simulink model "IEEE123_4subsystem"  (R2022b)
settings: Solver=ode4  StartTime=0.0  StopTime=inf  FixedStep=Ts  MaxStep=1e-4  RelTol=1e-3
PreLoadFcn:
  | Ts = 50e-6;
PostLoadFcn:
  | Ts = 50e-6;
InitFcn:
  | %%%%%%%%%%%%%%%%%%%%%%%%
  | % Simulation data for the IEEE 123 Node Test Feeder model
  | %%%%%%%%%%%%%%%%%%%%%%%
  | 
  | % miles/km
  | mi2km = 1.60934;
  | 
  | % feet to km
  | ft2km = 0.0003048;
  | 
  | % microsiemens to Farads
  | ms2F = 1/2/pi/60*1e-6;
  | 
  | %% Configuration 1 - series reactance - ohm/mile
  | 
  | R_1 = [0.4576 0.1560 0.1535;0.1560 0.4666 0.1580;0.1535 0.1580 0.4615];
  | X_1 = [1.0780 0.5017 0.3849;0.5017 1.0482 0.4236;0.3849 0.4236 1.0651];
  | 
  | % charging susceptance - microsiemens/mile
  | 
  | B_1 = [5.6765 -1.8319 -0.6982;-1.8319 5.9809 -1.1645;-0.6982 -1.1645 5.3971];
  | 
  | % convert for SPS
  | 
  | R_1 = R_1/mi2km;
  | 
  | Rs_1=(R_1(1,1)+R_1(2,2)+R_1(3,3))/3;
  | Rm_1=(R_1(1,2)+R_1(1,3)+R_1(2,3))/3;
  | R1_1=Rs_1-Rm_1;
  | R0_1=Rs_1+2*Rm_1;
  | 
  | L_1 = X_1/mi2km/2/pi/60;
  | 
  | Ls_1=(L_1(1,1)+L_1(2,2)+L_1(3,3))/3;
  | Lm_1=(L_1(1,2)+L_1(1,3)+L_1(2,3))/3;
  | L1_1=Ls_1-Lm_1;
  | L0_1=Ls_1+2*Lm_1;
  | 
  | C_1 = B_1/mi2km*ms2F;
  | 
  | Cs_1=(C_1(1,1)+C_1(2,2)+C_1(3,3))/3;
  | Cm_1=(C_1(1,2)+C_1(1,3)+C_1(2,3))/3;
  | C1_1=Cs_1-Cm_1;
  | C0_1=Cs_1+2*Cm_1;
  | 
  | 
  | %% Configuration 2 - series reactance - ohm/mile
  | 
  | R_2 = [0.4666 0.1580 0.1560;0.1580 0.4615 0.1535;0.1560 0.1535 0.4576];
  | X_2 = [1.0482 0.4236 0.5017;0.4236 1.0651 0.3849;0.5017 0.3849 1.0780];
  | 
  | % charging susceptance - microsiemens/mile
  | 
  | B_2 = [5.9809 -1.1645 -1.8319;-1.1645 5.3971 -0.6982;-1.8319 -0.6982 5.6765];
  | 
  | % convert for SPS
  | 
  | R_2 = R_2/mi2km;
  | 
  | Rs_2=(R_2(1,1)+R_2(2,2)+R_2(3,3))/3;
  | ... (+341 lines)
undefined symbols (not defined in the file): D1, Delta, find_system, I, Left, MOV_segment9, powergui, Right, type, V, X
libraries: spsGroundLib x242, spsThreePhaseVIMeasurementLib x134, spsSeriesRLCBranchLib x107, spsSeriesRLCLoadLib x83, spsPiSectionLineLib x61, spsThreePhasePISectionLineLib x60, spsVoltageMeasurementLib x52, spsDCVoltageSourceLib x36, ssn_lib x28, artemis x24, spsACCurrentSourceLib x18, spsOnDelayLib x18
(part 4 of 15)

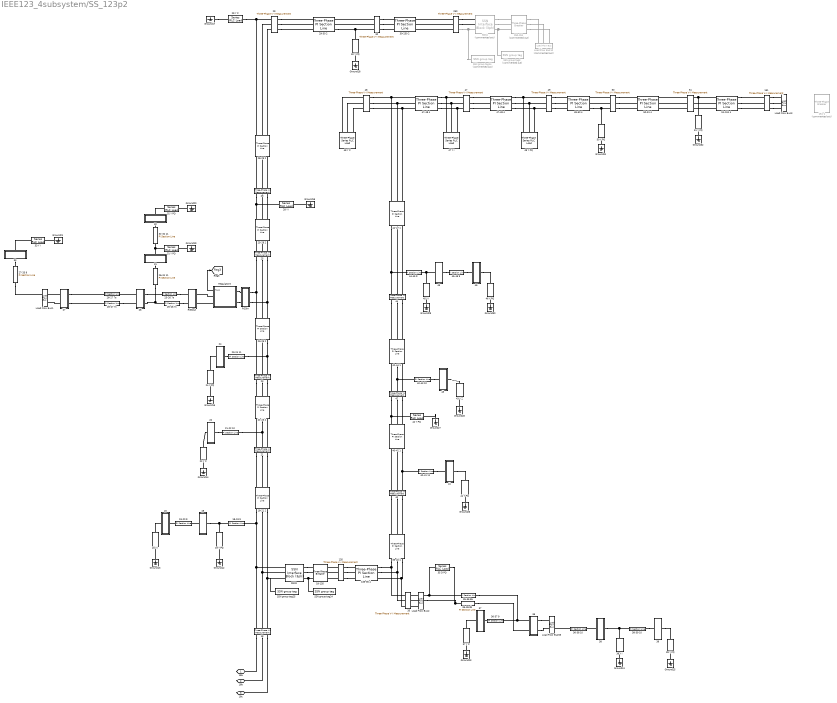
== system IEEE123_4subsystem/SS_123p2 ==
  135 : spsThreePhaseVIMeasurementLib/Three-Phase V-I Measurement  VoltageMeasurement=phase-to-ground  SetLabelV=on  LabelV=V135  Vpu=off  VpuLL=off  CurrentMeasurement=no  SetLabelI=on  LabelI=I800  Ipu=off  Pbase=100e6  Vbase=24900  OutputType=Complex  PhasorSimulation=off  PSBequivalent=0
  135-35 4 : spsThreePhasePISectionLineLib/Three-Phase PI Section Line  LConnTagsString=a|b|c  RConnTagsString=A|B|C  Length=375*ft2km  Frequency=60  Resistances=[R1_4 R0_4]  Inductances=[L1_4 L0_4]  Capacitances=[C1_4 C0_4]
  151 : spsThreePhaseVIMeasurementLib/Three-Phase V-I Measurement  VoltageMeasurement=phase-to-ground  SetLabelV=on  LabelV=V151  Vpu=off  VpuLL=off  CurrentMeasurement=no  SetLabelI=on  LabelI=I65  Ipu=off  Pbase=100e6  Vbase=24900  OutputType=Complex  PhasorSimulation=off  PSBequivalent=0
  151-1 : spsThreePhaseBreakerLib/Three-Phase Breaker  Commented=on  InitialState=open  SwitchA=on  SwitchB=on  SwitchC=on  SwitchTimes="[1/60  5/60]"  External=off  BreakerResistance=0.01  SnubberResistance=1e6  SnubberCapacitance=inf  Measurements=None
  18 : spsThreePhaseVIMeasurementLib/Three-Phase V-I Measurement  VoltageMeasurement=phase-to-ground  SetLabelV=on  LabelV=V18  Vpu=off  VpuLL=off  CurrentMeasurement=yes  SetLabelI=on  LabelI=I18  Ipu=off  Pbase=100e6  Vbase=24900  OutputType=Complex  PhasorSimulation=off  PSBequivalent=0
  18-135 : spsThreePhaseBreakerLib/Three-Phase Breaker  InitialState=closed  SwitchA=on  SwitchB=on  SwitchC=on  SwitchTimes="[1/60  5/60]"  External=off  BreakerResistance=0.01  SnubberResistance=1e6  SnubberCapacitance=inf  Measurements=None
  18-19 9 : spsPiSectionLineLib/Pi Section Line  LConnTagsString=__new0  RConnTagsString=__new0  Phases=1  PiSections=1  Length=250*ft2km  Frequency=60  Resistance=R1_9  Inductance=L1_9  Capacitance=C1_9  SpecifyConductance=off  Conductance=0  Measurements=None  Measurements2=None
      settings: LibrarySourceBlock=sps_lib/Power Grid Elements/Pi Section Line
  18-21 2 : spsThreePhasePISectionLineLib/Three-Phase PI Section Line  LConnTagsString=a|b|c  RConnTagsString=A|B|C  Length=300*ft2km  Frequency=60  Resistances=[R1_2 R0_2]  Inductances=[L1_2 L0_2]  Capacitances=[C1_2 C0_2]
  19 : Subsystem
  19 Y PQ : spsSeriesRLCLoadLib/Series RLC Load  LConnTagsString=a  RConnTagsString=__new0  NominalVoltage=1.0*2401.78  NominalFrequency=60  ActivePower=40e3  InductivePower=20e3  CapacitivePower=0  Setx0=off  InitialVoltage=0  SetiL0=off  InitialCurrent=0  Measurements=None  LoadType=constant PQ
  19-20 9 : spsPiSectionLineLib/Pi Section Line  LConnTagsString=__new0  RConnTagsString=__new0  Phases=1  PiSections=1  Length=325*ft2km  Frequency=60  Resistance=R1_9  Inductance=L1_9  Capacitance=C1_9  SpecifyConductance=off  Conductance=0  Measurements=None  Measurements2=None
      settings: LibrarySourceBlock=sps_lib/Power Grid Elements/Pi Section Line
  20 : Subsystem
  20 Y I : spsSeriesRLCLoadLib/Series RLC Load  LConnTagsString=a  RConnTagsString=__new0  NominalVoltage=1.0*2401.78  NominalFrequency=60  ActivePower=40e3  InductivePower=20e3  CapacitivePower=0  Setx0=off  InitialVoltage=0  SetiL0=off  InitialCurrent=0  Measurements=None  LoadType=constant I
  21 : spsThreePhaseVIMeasurementLib/Three-Phase V-I Measurement  VoltageMeasurement=phase-to-ground  SetLabelV=on  LabelV=V21  Vpu=off  VpuLL=off  CurrentMeasurement=yes  SetLabelI=on  LabelI=I21  Ipu=off  Pbase=100e6  Vbase=24900  OutputType=Complex  PhasorSimulation=off  PSBequivalent=0
  21-22 10 : spsPiSectionLineLib/Pi Section Line  LConnTagsString=__new0  RConnTagsString=__new0  Phases=1  PiSections=1  Length=525*ft2km  Frequency=60  Resistance=R1_10  Inductance=L1_10  Capacitance=C1_10  SpecifyConductance=off  Conductance=0  Measurements=None  Measurements2=None
      settings: LibrarySourceBlock=sps_lib/Power Grid Elements/Pi Section Line
  21-23 2 : spsThreePhasePISectionLineLib/Three-Phase PI Section Line  LConnTagsString=a|b|c  RConnTagsString=A|B|C  Length=250*ft2km  Frequency=60  Resistances=[R1_2 R0_2]  Inductances=[L1_2 L0_2]  Capacitances=[C1_2 C0_2]
  22 : Subsystem
  22 Y Z : spsSeriesRLCLoadLib/Series RLC Load  LConnTagsString=a  RConnTagsString=__new0  NominalVoltage=1.0*2401.78  NominalFrequency=60  ActivePower=40e3  InductivePower=20e3  CapacitivePower=0  Setx0=off  InitialVoltage=0  SetiL0=off  InitialCurrent=0  Measurements=None  LoadType=constant Z
  23 : spsThreePhaseVIMeasurementLib/Three-Phase V-I Measurement  VoltageMeasurement=phase-to-ground  SetLabelV=on  LabelV=V23  Vpu=off  VpuLL=off  CurrentMeasurement=no  SetLabelI=on  LabelI=I800  Ipu=off  Pbase=100e6  Vbase=24900  OutputType=Complex  PhasorSimulation=off  PSBequivalent=0
  23-24 11 : spsPiSectionLineLib/Pi Section Line  LConnTagsString=__new0  RConnTagsString=__new0  Phases=1  PiSections=1  Length=550*ft2km  Frequency=60  Resistance=R1_11  Inductance=L1_11  Capacitance=C1_11  SpecifyConductance=off  Conductance=0  Measurements=None  Measurements2=None
      settings: LibrarySourceBlock=sps_lib/Power Grid Elements/Pi Section Line
  23-25 2 : spsThreePhasePISectionLineLib/Three-Phase PI Section Line  LConnTagsString=a|b|c  RConnTagsString=A|B|C  Length=275*ft2km  Frequency=60  Resistances=[R1_2 R0_2]  Inductances=[L1_2 L0_2]  Capacitances=[C1_2 C0_2]
  24 : Subsystem
  24 Y PQ : spsSeriesRLCLoadLib/Series RLC Load  LConnTagsString=a  RConnTagsString=__new0  NominalVoltage=1.0*2401.78  NominalFrequency=60  ActivePower=40e3  InductivePower=20e3  CapacitivePower=0  Setx0=off  InitialVoltage=0  SetiL0=off  InitialCurrent=0  Measurements=None  LoadType=constant PQ
  25 : spsThreePhaseVIMeasurementLib/Three-Phase V-I Measurement  VoltageMeasurement=phase-to-ground  SetLabelV=on  LabelV=V25  Vpu=off  VpuLL=off  CurrentMeasurement=no  SetLabelI=on  LabelI=I800  Ipu=off  Pbase=100e6  Vbase=24900  OutputType=Complex  PhasorSimulation=off  PSBequivalent=0
  25-26 7a : spsPiSectionLineLib/Pi Section Line  LConnTagsString=__new0  RConnTagsString=__new0  Phases=1  PiSections=1  Length=350*ft2km  Frequency=60  Resistance=R1_7  Inductance=L1_7  Capacitance=C1_7  SpecifyConductance=off  Conductance=0  Measurements=None  Measurements2=None
      settings: LibrarySourceBlock=sps_lib/Power Grid Elements/Pi Section Line
  25-26 7c : spsPiSectionLineLib/Pi Section Line  LConnTagsString=__new0  RConnTagsString=__new0  Phases=1  PiSections=1  Length=350*ft2km  Frequency=60  Resistance=R1_7  Inductance=L1_7  Capacitance=C1_7  SpecifyConductance=off  Conductance=0  Measurements=None  Measurements2=None
      settings: LibrarySourceBlock=sps_lib/Power Grid Elements/Pi Section Line
  25-28 2 : spsThreePhasePISectionLineLib/Three-Phase PI Section Line  LConnTagsString=a|b|c  RConnTagsString=A|B|C  Length=200*ft2km  Frequency=60  Resistances=[R1_2 R0_2]  Inductances=[L1_2 L0_2]  Capacitances=[C1_2 C0_2]
  250 : spsThreePhaseVIMeasurementLib/Three-Phase V-I Measurement  VoltageMeasurement=phase-to-ground  SetLabelV=on  LabelV=V250  Vpu=off  VpuLL=off  CurrentMeasurement=no  SetLabelI=on  LabelI=I800  Ipu=off  Pbase=100e6  Vbase=24900  OutputType=Complex  PhasorSimulation=off  PSBequivalent=0
  250-251 : spsThreePhaseBreakerLib/Three-Phase Breaker  Commented=on  InitialState=open  SwitchA=on  SwitchB=on  SwitchC=on  SwitchTimes="[1/60  5/60]"  External=off  BreakerResistance=0.01  SnubberResistance=1e6  SnubberCapacitance=inf  Measurements=None
  26 : Subsystem
  26-27 7a : spsPiSectionLineLib/Pi Section Line  LConnTagsString=__new0  RConnTagsString=__new0  Phases=1  PiSections=1  Length=275*ft2km  Frequency=60  Resistance=R1_7  Inductance=L1_7  Capacitance=C1_7  SpecifyConductance=off  Conductance=0  Measurements=None  Measurements2=None
      settings: LibrarySourceBlock=sps_lib/Power Grid Elements/Pi Section Line
  26-27 7c : spsPiSectionLineLib/Pi Section Line  LConnTagsString=__new0  RConnTagsString=__new0  Phases=1  PiSections=1  Length=275*ft2km  Frequency=60  Resistance=R1_7  Inductance=L1_7  Capacitance=C1_7  SpecifyConductance=off  Conductance=0  Measurements=None  Measurements2=None
      settings: LibrarySourceBlock=sps_lib/Power Grid Elements/Pi Section Line
  26-31 11 : spsPiSectionLineLib/Pi Section Line  LConnTagsString=__new0  RConnTagsString=__new0  Phases=1  PiSections=1  Length=225*ft2km  Frequency=60  Resistance=R1_11  Inductance=L1_11  Capacitance=C1_11  SpecifyConductance=off  Conductance=0  Measurements=None  Measurements2=None
      settings: LibrarySourceBlock=sps_lib/Power Grid Elements/Pi Section Line
  27 : Subsystem
  27-33 9 : spsPiSectionLineLib/Pi Section Line  LConnTagsString=__new0  RConnTagsString=__new0  Phases=1  PiSections=1  Length=500*ft2km  Frequency=60  Resistance=R1_9  Inductance=L1_9  Capacitance=C1_9  SpecifyConductance=off  Conductance=0  Measurements=None  Measurements2=None
      settings: LibrarySourceBlock=sps_lib/Power Grid Elements/Pi Section Line
  28 : spsThreePhaseVIMeasurementLib/Three-Phase V-I Measurement  VoltageMeasurement=phase-to-ground  SetLabelV=on  LabelV=V28  Vpu=off  VpuLL=off  CurrentMeasurement=no  SetLabelI=on  LabelI=I800  Ipu=off  Pbase=100e6  Vbase=24900  OutputType=Complex  PhasorSimulation=off  PSBequivalent=0
  28 Y I : spsSeriesRLCLoadLib/Series RLC Load  LConnTagsString=a  RConnTagsString=__new0  NominalVoltage=1.0*2401.78  NominalFrequency=60  ActivePower=40e3  InductivePower=20e3  CapacitivePower=0  Setx0=off  InitialVoltage=0  SetiL0=off  InitialCurrent=0  Measurements=None  LoadType=constant I
  28-29 2 : spsThreePhasePISectionLineLib/Three-Phase PI Section Line  LConnTagsString=a|b|c  RConnTagsString=A|B|C  Length=300*ft2km  Frequency=60  Resistances=[R1_2 R0_2]  Inductances=[L1_2 L0_2]  Capacitances=[C1_2 C0_2]
  29 : spsThreePhaseVIMeasurementLib/Three-Phase V-I Measurement  VoltageMeasurement=phase-to-ground  SetLabelV=on  LabelV=V29  Vpu=off  VpuLL=off  CurrentMeasurement=no  SetLabelI=on  LabelI=I800  Ipu=off  Pbase=100e6  Vbase=24900  OutputType=Complex  PhasorSimulation=off  PSBequivalent=0
  29 Y Z : spsSeriesRLCLoadLib/Series RLC Load  LConnTagsString=a  RConnTagsString=__new0  NominalVoltage=1.0*2401.78  NominalFrequency=60  ActivePower=40e3  InductivePower=20e3  CapacitivePower=0  Setx0=off  InitialVoltage=0  SetiL0=off  InitialCurrent=0  Measurements=None  LoadType=constant Z
  29-30 2 : spsThreePhasePISectionLineLib/Three-Phase PI Section Line  LConnTagsString=a|b|c  RConnTagsString=A|B|C  Length=350*ft2km  Frequency=60  Resistances=[R1_2 R0_2]  Inductances=[L1_2 L0_2]  Capacitances=[C1_2 C0_2]
  "30 " : spsThreePhaseVIMeasurementLib/Three-Phase V-I Measurement  VoltageMeasurement=phase-to-ground  SetLabelV=on  LabelV=V30  Vpu=off  VpuLL=off  CurrentMeasurement=no  SetLabelI=on  LabelI=I800  Ipu=off  Pbase=100e6  Vbase=24900  OutputType=Complex  PhasorSimulation=off  PSBequivalent=0
  30 Y PQ : spsSeriesRLCLoadLib/Series RLC Load  LConnTagsString=a  RConnTagsString=__new0  NominalVoltage=1.0*2401.78  NominalFrequency=60  ActivePower=40e3  InductivePower=20e3  CapacitivePower=0  Setx0=off  InitialVoltage=0  SetiL0=off  InitialCurrent=0  Measurements=None  LoadType=constant PQ
  30-250 2 : spsThreePhasePISectionLineLib/Three-Phase PI Section Line  LConnTagsString=a|b|c  RConnTagsString=A|B|C  Length=200*ft2km  Frequency=60  Resistances=[R1_2 R0_2]  Inductances=[L1_2 L0_2]  Capacitances=[C1_2 C0_2]
  31 : Subsystem
  31 Y PQ : spsSeriesRLCLoadLib/Series RLC Load  LConnTagsString=a  RConnTagsString=__new0  NominalVoltage=1.0*2401.78  NominalFrequency=60  ActivePower=20e3  InductivePower=10e3  CapacitivePower=0  Setx0=off  InitialVoltage=0  SetiL0=off  InitialCurrent=0  Measurements=None  LoadType=constant PQ
  31-32 11 : spsPiSectionLineLib/Pi Section Line  LConnTagsString=__new0  RConnTagsString=__new0  Phases=1  PiSections=1  Length=300*ft2km  Frequency=60  Resistance=R1_11  Inductance=L1_11  Capacitance=C1_11  SpecifyConductance=off  Conductance=0  Measurements=None  Measurements2=None
      settings: LibrarySourceBlock=sps_lib/Power Grid Elements/Pi Section Line
  32 : Subsystem
  32 Y PQ : spsSeriesRLCLoadLib/Series RLC Load  LConnTagsString=a  RConnTagsString=__new0  NominalVoltage=1.0*2401.78  NominalFrequency=60  ActivePower=20e3  InductivePower=10e3  CapacitivePower=0  Setx0=off  InitialVoltage=0  SetiL0=off  InitialCurrent=0  Measurements=None  LoadType=constant PQ
  33 : Subsystem
  33 Y I : spsSeriesRLCLoadLib/Series RLC Load  LConnTagsString=a  RConnTagsString=__new0  NominalVoltage=1.0*2401.78  NominalFrequency=60  ActivePower=40e3  InductivePower=20e3  CapacitivePower=0  Setx0=off  InitialVoltage=0  SetiL0=off  InitialCurrent=0  Measurements=None  LoadType=constant I
  35 : spsThreePhaseVIMeasurementLib/Three-Phase V-I Measurement  VoltageMeasurement=phase-to-ground  SetLabelV=on  LabelV=V35  Vpu=off  VpuLL=off  CurrentMeasurement=no  SetLabelI=on  LabelI=I800  Ipu=off  Pbase=100e6  Vbase=24900  OutputType=Complex  PhasorSimulation=off  PSBequivalent=0
  35 D PQ : spsSeriesRLCLoadLib/Series RLC Load  LConnTagsString=a  RConnTagsString=__new0  NominalVoltage=1.0*4160  NominalFrequency=60  ActivePower=40e3  InductivePower=20e3  CapacitivePower=0  Setx0=off  InitialVoltage=0  SetiL0=off  InitialCurrent=0  Measurements=None  LoadType=constant I
  35-36 8a : spsPiSectionLineLib/Pi Section Line  LConnTagsString=__new0  RConnTagsString=__new0  Phases=1  PiSections=1  Length=650*ft2km  Frequency=60  Resistance=R1_8  Inductance=L1_8  Capacitance=C1_8  SpecifyConductance=off  Conductance=0  Measurements=None  Measurements2=None
      settings: LibrarySourceBlock=sps_lib/Power Grid Elements/Pi Section Line
  35-36 8b : spsPiSectionLineLib/Pi Section Line  LConnTagsString=__new0  RConnTagsString=__new0  Phases=1  PiSections=1  Length=650*ft2km  Frequency=60  Resistance=R1_8  Inductance=L1_8  Capacitance=C1_8  SpecifyConductance=off  Conductance=0  Measurements=None  Measurements2=None
      settings: LibrarySourceBlock=sps_lib/Power Grid Elements/Pi Section Line
  35-40 1 : spsThreePhasePISectionLineLib/Three-Phase PI Section Line  LConnTagsString=a|b|c  RConnTagsString=A|B|C  Length=250*ft2km  Frequency=60  Resistances=[R1_1 R0_1]  Inductances=[L1_1 L0_1]  Capacitances=[C1_1 C0_1]
  36 : Subsystem
  36-37 9 : spsPiSectionLineLib/Pi Section Line  LConnTagsString=__new0  RConnTagsString=__new0  Phases=1  PiSections=1  Length=300*ft2km  Frequency=60  Resistance=R1_9  Inductance=L1_9  Capacitance=C1_9  SpecifyConductance=off  Conductance=0  Measurements=None  Measurements2=None
      settings: LibrarySourceBlock=sps_lib/Power Grid Elements/Pi Section Line
  36-38 10 : spsPiSectionLineLib/Pi Section Line  LConnTagsString=__new0  RConnTagsString=__new0  Phases=1  PiSections=1  Length=250*ft2km  Frequency=60  Resistance=R1_10  Inductance=L1_10  Capacitance=C1_10  SpecifyConductance=off  Conductance=0  Measurements=None  Measurements2=None
      settings: LibrarySourceBlock=sps_lib/Power Grid Elements/Pi Section Line
  37 : Subsystem
  37 Y Z : spsSeriesRLCLoadLib/Series RLC Load  LConnTagsString=a  RConnTagsString=__new0  NominalVoltage=1.0*2401.78  NominalFrequency=60  ActivePower=40e3  InductivePower=20e3  CapacitivePower=0  Setx0=off  InitialVoltage=0  SetiL0=off  InitialCurrent=0  Measurements=None  LoadType=constant Z
  38 : Subsystem
  38 Y I : spsSeriesRLCLoadLib/Series RLC Load  LConnTagsString=a  RConnTagsString=__new0  NominalVoltage=1.0*2401.78  NominalFrequency=60  ActivePower=20e3  InductivePower=10e3  CapacitivePower=0  Setx0=off  InitialVoltage=0  SetiL0=off  InitialCurrent=0  Measurements=None  LoadType=constant I
  38-39 10 : spsPiSectionLineLib/Pi Section Line  LConnTagsString=__new0  RConnTagsString=__new0  Phases=1  PiSections=1  Length=325*ft2km  Frequency=60  Resistance=R1_10  Inductance=L1_10  Capacitance=C1_10  SpecifyConductance=off  Conductance=0  Measurements=None  Measurements2=None
      settings: LibrarySourceBlock=sps_lib/Power Grid Elements/Pi Section Line
  39 : Subsystem
  39 Y PQ : spsSeriesRLCLoadLib/Series RLC Load  LConnTagsString=a  RConnTagsString=__new0  NominalVoltage=1.0*2401.78  NominalFrequency=60  ActivePower=20e3  InductivePower=10e3  CapacitivePower=0  Setx0=off  InitialVoltage=0  SetiL0=off  InitialCurrent=0  Measurements=None  LoadType=constant PQ
  40 : spsThreePhaseVIMeasurementLib/Three-Phase V-I Measurement  VoltageMeasurement=phase-to-ground  SetLabelV=on  LabelV=V40  Vpu=off  VpuLL=off  CurrentMeasurement=no  SetLabelI=on  LabelI=I800  Ipu=off  Pbase=100e6  Vbase=24900  OutputType=Complex  PhasorSimulation=off  PSBequivalent=0
  40-41 11 : spsPiSectionLineLib/Pi Section Line  LConnTagsString=__new0  RConnTagsString=__new0  Phases=1  PiSections=1  Length=325*ft2km  Frequency=60  Resistance=R1_11  Inductance=L1_11  Capacitance=C1_11  SpecifyConductance=off  Conductance=0  Measurements=None  Measurements2=None
      settings: LibrarySourceBlock=sps_lib/Power Grid Elements/Pi Section Line
  40-42 1 : spsThreePhasePISectionLineLib/Three-Phase PI Section Line  LConnTagsString=a|b|c  RConnTagsString=A|B|C  Length=250*ft2km  Frequency=60  Resistances=[R1_1 R0_1]  Inductances=[L1_1 L0_1]  Capacitances=[C1_1 C0_1]
  41 : Subsystem
  41 Y PQ : spsSeriesRLCLoadLib/Series RLC Load  LConnTagsString=a  RConnTagsString=__new0  NominalVoltage=1.0*2401.78  NominalFrequency=60  ActivePower=20e3  InductivePower=10e3  CapacitivePower=0  Setx0=off  InitialVoltage=0  SetiL0=off  InitialCurrent=0  Measurements=None  LoadType=constant PQ
  42 : spsThreePhaseVIMeasurementLib/Three-Phase V-I Measurement  VoltageMeasurement=phase-to-ground  SetLabelV=on  LabelV=V42  Vpu=off  VpuLL=off  CurrentMeasurement=no  SetLabelI=on  LabelI=I800  Ipu=off  Pbase=100e6  Vbase=24900  OutputType=Complex  PhasorSimulation=off  PSBequivalent=0
  42 Y PQ : spsSeriesRLCLoadLib/Series RLC Load  LConnTagsString=a  RConnTagsString=__new0  NominalVoltage=1.0*2401.78  NominalFrequency=60  ActivePower=20e3  InductivePower=10e3  CapacitivePower=0  Setx0=off  InitialVoltage=0  SetiL0=off  InitialCurrent=0  Measurements=None  LoadType=constant PQ
  42-43 10 : spsPiSectionLineLib/Pi Section Line  LConnTagsString=__new0  RConnTagsString=__new0  Phases=1  PiSections=1  Length=500*ft2km  Frequency=60  Resistance=R1_10  Inductance=L1_10  Capacitance=C1_10  SpecifyConductance=off  Conductance=0  Measurements=None  Measurements2=None
      settings: LibrarySourceBlock=sps_lib/Power Grid Elements/Pi Section Line
  42-44 1 : spsThreePhasePISectionLineLib/Three-Phase PI Section Line  LConnTagsString=a|b|c  RConnTagsString=A|B|C  Length=200*ft2km  Frequency=60  Resistances=[R1_1 R0_1]  Inductances=[L1_1 L0_1]  Capacitances=[C1_1 C0_1]
  43 : Subsystem
  43 Y Z : spsSeriesRLCLoadLib/Series RLC Load  LConnTagsString=a  RConnTagsString=__new0  NominalVoltage=1.0*2401.78  NominalFrequency=60  ActivePower=40e3  InductivePower=20e3  CapacitivePower=0  Setx0=off  InitialVoltage=0  SetiL0=off  InitialCurrent=0  Measurements=None  LoadType=constant Z
  44 : spsThreePhaseVIMeasurementLib/Three-Phase V-I Measurement  VoltageMeasurement=phase-to-ground  SetLabelV=on  LabelV=V44  Vpu=off  VpuLL=off  CurrentMeasurement=no  SetLabelI=on  LabelI=I800  Ipu=off  Pbase=100e6  Vbase=24900  OutputType=Complex  PhasorSimulation=off  PSBequivalent=0
  44-45 9 : spsPiSectionLineLib/Pi Section Line  LConnTagsString=__new0  RConnTagsString=__new0  Phases=1  PiSections=1  Length=200*ft2km  Frequency=60  Resistance=R1_9  Inductance=L1_9  Capacitance=C1_9  SpecifyConductance=off  Conductance=0  Measurements=None  Measurements2=None
      settings: LibrarySourceBlock=sps_lib/Power Grid Elements/Pi Section Line
  44-47 1 : spsThreePhasePISectionLineLib/Three-Phase PI Section Line  LConnTagsString=a|b|c  RConnTagsString=A|B|C  Length=250*ft2km  Frequency=60  Resistances=[R1_1 R0_1]  Inductances=[L1_1 L0_1]  Capacitances=[C1_1 C0_1]
  45 : Subsystem
  45 Y I : spsSeriesRLCLoadLib/Series RLC Load  LConnTagsString=a  RConnTagsString=__new0  NominalVoltage=1.0*2401.78  NominalFrequency=60  ActivePower=20e3  InductivePower=10e3  CapacitivePower=0  Setx0=off  InitialVoltage=0  SetiL0=off  InitialCurrent=0  Measurements=None  LoadType=constant I
  45-46 9 : spsPiSectionLineLib/Pi Section Line  LConnTagsString=__new0  RConnTagsString=__new0  Phases=1  PiSections=1  Length=300*ft2km  Frequency=60  Resistance=R1_9  Inductance=L1_9  Capacitance=C1_9  SpecifyConductance=off  Conductance=0  Measurements=None  Measurements2=None
      settings: LibrarySourceBlock=sps_lib/Power Grid Elements/Pi Section Line
  46 : Subsystem
  46 Y PQ : spsSeriesRLCLoadLib/Series RLC Load  LConnTagsString=a  RConnTagsString=__new0  NominalVoltage=1.0*2401.78  NominalFrequency=60  ActivePower=20e3  InductivePower=10e3  CapacitivePower=0  Setx0=off  InitialVoltage=0  SetiL0=off  InitialCurrent=0  Measurements=None  LoadType=constant PQ
  47 : spsThreePhaseVIMeasurementLib/Three-Phase V-I Measurement  VoltageMeasurement=phase-to-ground  SetLabelV=on  LabelV=V47  Vpu=off  VpuLL=off  CurrentMeasurement=no  SetLabelI=on  LabelI=I800  Ipu=off  Pbase=100e6  Vbase=24900  OutputType=Complex  PhasorSimulation=off  PSBequivalent=0
  47 Y I : spsThreePhaseSeriesRLCLoadLib/Three-Phase Series RLC Load  LConnTagsString=A|B|C  Configuration=Y (grounded)  NominalVoltage=120e3  Vabc=[ 1.0 1.0 1.0]*2401.78  Vabcp=[1e3 1e3 1e3]  NominalFrequency=60  UnbalancedPower=on  ActivePower=1e+006  InductivePower=0  CapacitivePower=0  Pabc=[35 35 35 ]*1e3  QLabc=[25 25 25 ]*1e3  QCabc=[0 0 0]  Pabcp=[10e3 9e3 11e3]  QLabcp=[100 90 110]  QCabcp=[100 90 110]  Measurements=None  LoadType=constant I
  47-48 4 : spsThreePhasePISectionLineLib/Three-Phase PI Section Line  LConnTagsString=a|b|c  RConnTagsString=A|B|C  Length=150*ft2km  Frequency=60  Resistances=[R1_4 R0_4]  Inductances=[L1_4 L0_4]  Capacitances=[C1_4 C0_4]
  47-49 4 : spsThreePhasePISectionLineLib/Three-Phase PI Section Line  LConnTagsString=a|b|c  RConnTagsString=A|B|C  Length=250*ft2km  Frequency=60  Resistances=[R1_4 R0_4]  Inductances=[L1_4 L0_4]  Capacitances=[C1_4 C0_4]
  48 : spsThreePhaseVIMeasurementLib/Three-Phase V-I Measurement  VoltageMeasurement=phase-to-ground  SetLabelV=on  LabelV=V48  Vpu=off  VpuLL=off  CurrentMeasurement=no  SetLabelI=on  LabelI=I800  Ipu=off  Pbase=100e6  Vbase=24900  OutputType=Complex  PhasorSimulation=off  PSBequivalent=0
  48 Y Z : spsThreePhaseSeriesRLCLoadLib/Three-Phase Series RLC Load  LConnTagsString=A|B|C  Configuration=Y (grounded)  NominalVoltage=120e3  Vabc=[ 1.0 1.0 1.0]*2401.78  Vabcp=[1e3 1e3 1e3]  NominalFrequency=60  UnbalancedPower=on  ActivePower=1e+006  InductivePower=0  CapacitivePower=0  Pabc=[70 70 70]*1e3  QLabc=[50 50 50]*1e3  QCabc=[0 0 0]  Pabcp=[10e3 9e3 11e3]  QLabcp=[100 90 110]  QCabcp=[100 90 110]  Measurements=None  LoadType=constant Z
  49 : spsThreePhaseVIMeasurementLib/Three-Phase V-I Measurement  VoltageMeasurement=phase-to-ground  SetLabelV=on  LabelV=V49  Vpu=off  VpuLL=off  CurrentMeasurement=no  SetLabelI=on  LabelI=I800  Ipu=off  Pbase=100e6  Vbase=24900  OutputType=Complex  PhasorSimulation=off  PSBequivalent=0
  49 Y PQ : spsThreePhaseSeriesRLCLoadLib/Three-Phase Series RLC Load  LConnTagsString=A|B|C  Configuration=Y (grounded)  NominalVoltage=120e3  Vabc=[ 1.0 1.0 1.0]*2401.78  Vabcp=[1e3 1e3 1e3]  NominalFrequency=60  UnbalancedPower=on  ActivePower=1e+006  InductivePower=0  CapacitivePower=0  Pabc=[35 70 35]*1e3  QLabc=[25 50 20]*1e3  QCabc=[0 0 0]  Pabcp=[10e3 9e3 11e3]  QLabcp=[100 90 110]  QCabcp=[100 90 110]  Measurements=None  LoadType=constant PQ
  49-50 4 : spsThreePhasePISectionLineLib/Three-Phase PI Section Line  LConnTagsString=a|b|c  RConnTagsString=A|B|C  Length=250*ft2km  Frequency=60  Resistances=[R1_4 R0_4]  Inductances=[L1_4 L0_4]  Capacitances=[C1_4 C0_4]
  50 : spsThreePhaseVIMeasurementLib/Three-Phase V-I Measurement  VoltageMeasurement=phase-to-ground  SetLabelV=on  LabelV=V50  Vpu=off  VpuLL=off  CurrentMeasurement=no  SetLabelI=on  LabelI=I800  Ipu=off  Pbase=100e6  Vbase=24900  OutputType=Complex  PhasorSimulation=off  PSBequivalent=0
  50 Y PQ : spsSeriesRLCLoadLib/Series RLC Load  LConnTagsString=a  RConnTagsString=__new0  NominalVoltage=1.0*2401.78  NominalFrequency=60  ActivePower=40e3  InductivePower=20e3  CapacitivePower=0  Setx0=off  InitialVoltage=0  SetiL0=off  InitialCurrent=0  Measurements=None  LoadType=constant PQ
  50-51 4 : spsThreePhasePISectionLineLib/Three-Phase PI Section Line  LConnTagsString=a|b|c  RConnTagsString=A|B|C  Length=250*ft2km  Frequency=60  Resistances=[R1_4 R0_4]  Inductances=[L1_4 L0_4]  Capacitances=[C1_4 C0_4]
  51 : spsThreePhaseVIMeasurementLib/Three-Phase V-I Measurement  VoltageMeasurement=phase-to-ground  SetLabelV=on  LabelV=V51  Vpu=off  VpuLL=off  CurrentMeasurement=no  SetLabelI=on  LabelI=I800  Ipu=off  Pbase=100e6  Vbase=24900  OutputType=Complex  PhasorSimulation=off  PSBequivalent=0
  51 Y PQ : spsSeriesRLCLoadLib/Series RLC Load  LConnTagsString=a  RConnTagsString=__new0  NominalVoltage=1.0*2401.78  NominalFrequency=60  ActivePower=20e3  InductivePower=10e3  CapacitivePower=0  Setx0=off  InitialVoltage=0  SetiL0=off  InitialCurrent=0  Measurements=None  LoadType=constant PQ
  51-151 4 : spsThreePhasePISectionLineLib/Three-Phase PI Section Line  LConnTagsString=a|b|c  RConnTagsString=A|B|C  Length=500*ft2km  Frequency=60  Resistances=[R1_4 R0_4]  Inductances=[L1_4 L0_4]  Capacitances=[C1_4 C0_4]
  Ground{12..21,23..32} (20 alike) : spsGroundLib/Ground  LConnTagsString=a
  Load Flow Bus1 : spsLoadFlowBusLib/Load Flow Bus  LConnTagsString=a|b  RConnTagsString=a|b  Phases=AC  Connectors=on both sides  ID=27  Vbase=4160/sqrt(3)  Vref=[1.0 1.0]  Vangle=[0 120]  VLF=1  VLFb=1  VLFc=1  angleLF=0  angleLFb=0  angleLFc=0
  Load Flow Bus10 : spsLoadFlowBusLib/Load Flow Bus  Commented=on  LConnTagsString=a|b|c  Phases=ABC  Connectors=on one side  ID=251  Vbase=4160/sqrt(3)  Vref=[1.0 1.0 1.0]  Vangle=[0 -120 120]  VLF=1  VLFb=1  VLFc=1  angleLF=0  angleLFb=0  angleLFc=0
  Load Flow Bus2 : spsLoadFlowBusLib/Load Flow Bus  LConnTagsString=a|b|c  RConnTagsString=a|b|c  Phases=ABC  Connectors=on both sides  ID=36  Vbase=4160/sqrt(3)  Vref=[1.0 1.0]  Vangle=[0 -120]  VLF=1  VLFb=1  VLFc=1  angleLF=0  angleLFb=0  angleLFc=0
  Load Flow Bus3 : spsLoadFlowBusLib/Load Flow Bus  LConnTagsString=a|b|c  Phases=ABC  Connectors=on one side  ID=150  Vbase=4160/sqrt(3)  Vref=[1.0 1.0 1.0]  Vangle=[0 -120 120]  VLF=1  VLFb=1  VLFc=1  angleLF=0  angleLFb=0  angleLFc=0
  Load Flow Bus55 : spsLoadFlowBusLib/Load Flow Bus  LConnTagsString=a|b  RConnTagsString=a|b  Phases=AB  Connectors=on both sides  ID=36  Vbase=4160/sqrt(3)  Vref=[1.0 1.0]  Vangle=[0 -120]  VLF=1  VLFb=1  VLFc=1  angleLF=0  angleLFb=0  angleLFc=0
  RG3in : Subsystem
  RG3out : Subsystem
  Regulator3 : Subsystem
  SSN group tag14 : artemis/SSN/SSN group tag  Commented=on  ssn_group_tag=ssn4a
  SSN group tag24 : artemis/SSN/SSN group tag  ssn_group_tag=ssn3b
  SSN group tag25 : artemis/SSN/SSN group tag  ssn_group_tag=ssn3a
  SSN group tag3 : artemis/SSN/SSN group tag  Commented=on  ssn_group_tag=ssn4b
  SSN3 : ssn_lib/SSN Interface Block (3ph)  nb_phase=3  nb_port=2  p1_type=I-type(Left)  p2_type=I-type(Right)  p3_type=V-type(Left)  p4_type=V-type(Left)  p5_type=V-type(Left)  p6_type=V-type(Left)  p7_type=V-type(Left)  p8_type=V-type(Left)  p9_type=V-type(Left)  p10_type=V-type(Left)  p11_type=V-type(Left)  p12_type=V-type(Left)  p13_type=V-type(Left)  p14_type=V-type(Left)  p15_type=V-type(Left)  p16_type=V-type(Left)  I_port_shunt_resistance=1e9
  SSN4 : ssn_lib/SSN Interface Block (3ph)  Commented=on  nb_phase=3  nb_port=2  p1_type=I-type(Left)  p2_type=I-type(Right)  p3_type=V-type(Left)  p4_type=V-type(Left)  p5_type=V-type(Left)  p6_type=V-type(Left)  p7_type=V-type(Left)  p8_type=V-type(Left)  p9_type=V-type(Left)  p10_type=V-type(Left)  p11_type=V-type(Left)  p12_type=V-type(Left)  p13_type=V-type(Left)  p14_type=V-type(Left)  p15_type=V-type(Left)  p16_type=V-type(Left)  I_port_shunt_resistance=1e9
  18a : PMIOPort  Side=Left
  18b : PMIOPort  Port=2  Side=Left
  18c : PMIOPort  Port=3  Side=Left
  tag scope: Reg3=global
  wires:
  Regulator3/1(Taps) -> [Reg3]
  connections:
  21/LConn1 -- 18-21 2/RConn1
  151/LConn3 -- Load Flow Bus3/LConn3
  19 Y PQ/LConn1 -- 19/LConn1 -- 18-19 9/RConn1
  21-22 10/LConn1 -- 21/RConn2 -- 21-23 2/LConn2
  135/RConn2 -- 135-35 4/LConn2
  50/LConn2 -- 49-50 4/RConn2
  42/LConn2 -- 40-42 1/RConn2
  44-45 9/LConn1 -- 44/RConn1 -- 44-47 1/LConn1
  SSN4/LConn3 -- 250/RConn3 -- SSN group tag14/LConn1
  32/LConn1 -- 31-32 11/RConn1
  Ground18/LConn1 -- 30 Y PQ/RConn1
  38 Y I/LConn1 -- 38/RConn1 -- 38-39 10/LConn1
  45 Y I/LConn1 -- 45/LConn1 -- 44-45 9/RConn1
  35-36 8a/RConn1 -- 36/LConn1 -- 36-37 9/LConn1
  48/LConn1 -- 48 Y Z/LConn1
  21/RConn1 -- 21-23 2/LConn1
  19/RConn1 -- 19-20 9/LConn1
  31 Y PQ/LConn1 -- 31/RConn1 -- 31-32 11/LConn1
  24/LConn1 -- 23-24 11/RConn1
  24 Y PQ/LConn1 -- 24/RConn1
  42/LConn3 -- 40-42 1/RConn3
  Ground29/LConn1 -- 45 Y I/RConn1
  51-151 4/RConn3 -- 151/RConn3
  "30 "/LConn2 -- 29-30 2/RConn2
  135/LConn1 -- 18-135/RConn1
  47/RConn1 -- 47-49 4/LConn1
  37 Y Z/LConn1 -- 37/RConn1
  49 Y PQ/LConn2 -- 49/LConn2 -- 47-49 4/RConn2
  40-41 11/LConn1 -- 40/RConn3 -- 40-42 1/LConn3
  51 Y PQ/LConn1 -- 51-151 4/LConn1 -- 51/RConn1
  50/RConn2 -- 50-51 4/LConn2
  Ground17/LConn1 -- 29 Y Z/RConn1
  250-251/RConn2 -- Load Flow Bus10/LConn2
  42/RConn1 -- 42-44 1/LConn1
  135-35 4/RConn2 -- 35/LConn2 -- 35-40 1/LConn2
  35 D PQ/LConn1 -- 35-36 8a/LConn1 -- Load Flow Bus2/RConn1
  40/LConn1 -- 35-40 1/RConn1
  23/RConn2 -- 23-25 2/LConn2
  22/LConn1 -- 21-22 10/RConn1
  51-151 4/LConn2 -- 51/RConn2
  50/LConn1 -- 49-50 4/RConn1
  50/RConn1 -- 50-51 4/LConn1
  23-24 11/LConn1 -- 23/RConn3 -- 23-25 2/LConn3
  36/RConn1 -- Load Flow Bus55/LConn1
  21/LConn3 -- 18-21 2/RConn3
  19-20 9/RConn1 -- 20/LConn1
  Ground30/LConn1 -- 46 Y PQ/RConn1
  28 Y I/LConn1 -- 28/LConn1 -- 25-28 2/RConn1
  SSN3/RConn2 -- 18-135/LConn2
  49 Y PQ/LConn1 -- 49/LConn1 -- 47-49 4/RConn1
  135/LConn2 -- 18-135/RConn2
  41/RConn1 -- 41 Y PQ/LConn1
  36-38 10/LConn1 -- Load Flow Bus55/RConn2
  28/RConn2 -- 28-29 2/LConn2
  47-48 4/LConn3 -- 48/RConn3 -- 44-47 1/RConn3
  29/RConn2 -- 29-30 2/LConn2
  50/RConn3 -- 50-51 4/LConn3
  Load Flow Bus2/LConn3 -- 35/RConn3
  250/LConn2 -- 30-250 2/RConn2
  37/LConn1 -- 36-37 9/RConn1
  42 Y PQ/LConn1 -- 42/LConn1 -- 40-42 1/RConn1
  28/RConn3 -- 28-29 2/LConn3
  Ground28/LConn1 -- 43 Y Z/RConn1
  Ground32/LConn1 -- 51 Y PQ/RConn1
  39/RConn1 -- 39 Y PQ/LConn1
  44/LConn1 -- 42-44 1/RConn1
  27/LConn2 -- 26-27 7c/LConn1
  26-27 7c/RConn1 -- 26/RConn2
  25-26 7c/RConn1 -- RG3out/RConn2
  25/LConn2 -- 23-25 2/RConn2
  33/LConn1 -- 27-33 9/RConn1
  Ground21/LConn1 -- 33 Y I/RConn1
  47 Y I/LConn3 -- 47/LConn3 -- 47-48 4/RConn3
  Regulator3/RConn1 -- RG3out/LConn1
  25/LConn1 -- RG3in/LConn1 -- 23-25 2/RConn1
  Regulator3/RConn2 -- RG3out/LConn2
  SSN4/RConn3 -- 250-251/LConn3 -- SSN group tag3/LConn1
  26-31 11/LConn1 -- 26/LConn2 -- 25-26 7c/LConn1
  49/RConn2 -- 49-50 4/LConn2
  42-43 10/RConn1 -- 43/LConn1
  250-251/RConn1 -- Load Flow Bus10/LConn1
  25-26 7a/RConn1 -- RG3out/RConn1
  "30 "/RConn1 -- 30-250 2/LConn1
  27/RConn2 -- Load Flow Bus1/RConn2
  42-43 10/LConn1 -- 42/RConn2 -- 42-44 1/LConn2
  40-41 11/RConn1 -- 41/LConn1
  Load Flow Bus2/LConn1 -- 35/RConn1
  Load Flow Bus2/LConn2 -- 35/RConn2
  151/LConn1 -- Load Flow Bus3/LConn1
  35-40 1/LConn3 -- 35/LConn3 -- 135-35 4/RConn3
  29/RConn3 -- 29-30 2/LConn3
  51-151 4/RConn2 -- 151/RConn2
  Ground20/LConn1 -- 32 Y PQ/RConn1
  151/LConn2 -- Load Flow Bus3/LConn2
  Regulator3/LConn1 -- RG3in/RConn1
  44/LConn2 -- 42-44 1/RConn2
  30 Y PQ/LConn1 -- "30 "/LConn3 -- 29-30 2/RConn3
  47-48 4/LConn1 -- 48/RConn1 -- 44-47 1/RConn1
  38-39 10/RConn1 -- 39/LConn1
  26/LConn1 -- 25-26 7a/LConn1
  Regulator3/LConn2 -- RG3in/RConn2
  25/RConn3 -- 25-28 2/LConn3
  21/LConn2 -- 18-21 2/RConn2
  33 Y I/LConn1 -- 33/RConn1
  135-35 4/RConn1 -- 35/LConn1 -- 35-40 1/LConn1
  48 Y Z/LConn2 -- 48/LConn2
  29/RConn1 -- 29-30 2/LConn1
  25/LConn3 -- RG3in/LConn2 -- 23-25 2/RConn3
  35 D PQ/RConn1 -- Load Flow Bus2/RConn2 -- 35-36 8b/LConn1
  27/LConn1 -- 26-27 7a/LConn1
  40/LConn2 -- 35-40 1/RConn2
  23/LConn3 -- 21-23 2/RConn3
  29/LConn2 -- 28-29 2/RConn2
  Ground16/LConn1 -- 28 Y I/RConn1
  135/RConn3 -- 135-35 4/LConn3
  23/LConn1 -- 21-23 2/RConn1
  43/RConn1 -- 43 Y Z/LConn1
  44/LConn3 -- 42-44 1/RConn3
  28-29 2/RConn1 -- 29/LConn1 -- 29 Y Z/LConn1
  Ground24/LConn1 -- 38 Y I/RConn1
  250/LConn1 -- 30-250 2/RConn1
  SSN3/RConn3 -- SSN group tag24/LConn1 -- 18-135/LConn3
  50 Y PQ/LConn1 -- 50/LConn3 -- 49-50 4/RConn3
  Ground19/LConn1 -- 31 Y PQ/RConn1
  250-251/RConn3 -- Load Flow Bus10/LConn3
  47 Y I/LConn2 -- 47/LConn2 -- 47-48 4/RConn2
  Ground15/LConn1 -- 24 Y PQ/RConn1
  29/LConn3 -- 28-29 2/RConn3
  51/LConn1 -- 50-51 4/RConn1
  SSN4/RConn1 -- 250-251/LConn1
  26/RConn1 -- 26-27 7a/RConn1
  250/LConn3 -- 30-250 2/RConn3
  40/LConn3 -- 35-40 1/RConn3
  28/LConn2 -- 25-28 2/RConn2
  18-21 2/LConn1 -- 18/RConn1 -- SSN3/LConn1 -- 18-19 9/LConn1
  250/RConn2 -- SSN4/LConn2
  44/RConn2 -- 44-47 1/LConn2
  46/RConn1 -- 46 Y PQ/LConn1
  18-21 2/LConn2 -- 18/RConn2 -- SSN3/LConn2
  49/RConn3 -- 49-50 4/LConn3
  51/LConn3 -- 50-51 4/RConn3
  250/RConn1 -- SSN4/LConn1
  18/LConn1 -- 18a/RConn1
  18-21 2/LConn3 -- 18/RConn3 -- SSN3/LConn3 -- SSN group tag25/LConn1
  45-46 9/RConn1 -- 46/LConn1
  "30 "/RConn2 -- 30-250 2/LConn2
  47 Y I/LConn1 -- 47/LConn1 -- 47-48 4/RConn1
  45/RConn1 -- 45-46 9/LConn1
  Ground12/LConn1 -- 19 Y PQ/RConn1
  51-151 4/RConn1 -- 151/RConn1
  20/RConn1 -- 20 Y I/LConn1
  51-151 4/LConn3 -- 51/RConn3
  27/RConn1 -- Load Flow Bus1/RConn1
  Ground26/LConn1 -- 41 Y PQ/RConn1
  23/LConn2 -- 21-23 2/RConn2
  23/RConn1 -- 23-25 2/LConn1
  22 Y Z/LConn1 -- 22/RConn1
  47/RConn3 -- 47-49 4/LConn3
  40/RConn2 -- 40-42 1/LConn2
  38/LConn1 -- 36-38 10/RConn1
  28/RConn1 -- 28-29 2/LConn1
  32 Y PQ/LConn1 -- 32/RConn1
  18/LConn2 -- 18b/RConn1
  35-36 8b/RConn1 -- 36/LConn2
  28/LConn3 -- 25-28 2/RConn3
  21/RConn3 -- 21-23 2/LConn3
  47-48 4/LConn2 -- 48/RConn2 -- 44-47 1/RConn2
  27-33 9/LConn1 -- Load Flow Bus1/LConn1
  31/LConn1 -- 26-31 11/RConn1
  Ground13/LConn1 -- 20 Y I/RConn1
  Ground31/LConn1 -- 50 Y PQ/RConn1
  Ground27/LConn1 -- 42 Y PQ/RConn1
  Ground25/LConn1 -- 39 Y PQ/RConn1
  Ground14/LConn1 -- 22 Y Z/RConn1
  Ground23/LConn1 -- 37 Y Z/RConn1
  135/RConn1 -- 135-35 4/LConn1
  SSN4/RConn2 -- 250-251/LConn2
  47/RConn2 -- 47-49 4/LConn2
  42/RConn3 -- 42-44 1/LConn3
  51/LConn2 -- 50-51 4/RConn2
  48/LConn3 -- 48 Y Z/LConn3
  "30 "/LConn1 -- 29-30 2/RConn1
  25/RConn1 -- 25-28 2/LConn1
  44/RConn3 -- 44-47 1/LConn3
  25/RConn2 -- 25-28 2/LConn2
  49 Y PQ/LConn3 -- 49/LConn3 -- 47-49 4/RConn3
  "30 "/RConn3 -- 30-250 2/LConn3
  135/LConn3 -- 18-135/RConn3
  SSN3/RConn1 -- 18-135/LConn1
  49/RConn1 -- 49-50 4/LConn1
  36/RConn2 -- Load Flow Bus55/LConn2
  40/RConn1 -- 40-42 1/LConn1
  18/LConn3 -- 18c/RConn1
